simulink model "lin_m_func"  (R2021a)
settings: Solver=VariableStepAuto  StartTime=0.0  StopTime=60.0  RelTol=1e-3
InitFcn:
  | start
values from neighbouring files (symbols this model uses):
  x0 = [0;0;0]    [start.m]
settings Model: Creator=mluser  LastModifiedBy=mluser

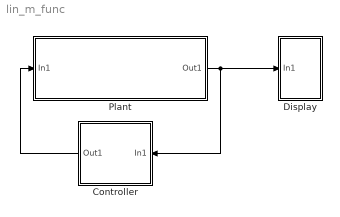
== system lin_m_func ==
  Controller : Subsystem
  Display : Subsystem
  Plant : Subsystem
  wires:
  Plant/1(Out1) -> Controller/1(In1), Display/1(In1)
  Controller/1(Out1) -> Plant/1(In1)

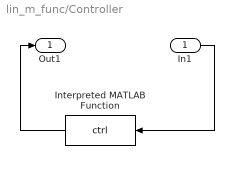
== system lin_m_func/Controller ==
  In1 : Inport
  Interpreted MATLAB Function : MATLABFcn  MATLABFcn=ctrl  OutputDimensions=1
  Out1 : Outport
  wires:
  In1/1 -> Interpreted MATLAB Function/1
  Interpreted MATLAB Function/1 -> Out1/1

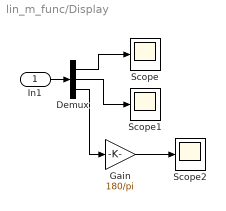
== system lin_m_func/Display ==
  In1 : Inport
  Demux : Demux  Outputs=3
  Gain : Gain  Gain=180/pi
  Scope : Scope
  Scope1 : Scope
  Scope2 : Scope
  wires:
  Demux/1 -> Scope/1
  Demux/3 -> Gain/1
  In1/1 -> Demux/1
  Demux/2 -> Scope1/1
  Gain/1 -> Scope2/1

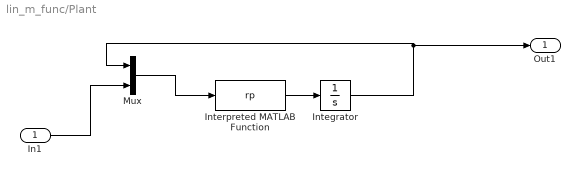
== system lin_m_func/Plant ==
  In1 : Inport
  Integrator : Integrator  InitialCondition=x0
  Interpreted MATLAB Function : MATLABFcn  MATLABFcn=rp  OutputDimensions=3
  Mux : Mux  Inputs=2
  Out1 : Outport
  wires:
  Mux/1 -> Interpreted MATLAB Function/1
  Interpreted MATLAB Function/1 -> Integrator/1
  In1/1 -> Mux/2
  Integrator/1 -> Out1/1, Mux/1
